simulink model "OpenLoopFreqResponse"  (R2015a)
settings: Solver=FixedStepDiscrete  SolverMode=SingleTasking  StartTime=0.0  StopTime=inf  FixedStep=Ts  RelTol=1e-3
InitFcn:
  | Ts = 0.010;
libraries: arduinolib x2, THLlib x2
settings Model: ExtModeTrigDuration=2  Creator=Carion  LastModifiedBy=SystemsUser
settings OptimizationCC: OptimizeModelRefInitCode=on  LifeSpan=1
settings DebuggingCC: UnderspecifiedInitializationDetection=Classic  MergeDetectMultiDrivingBlocksExec=none  StateNameClashWarn=warning
settings HardwareCC: ProdBitPerInt=16  ProdBitPerPointer=8  ProdIntDivRoundTo=Zero  ProdEndianess=LittleEndian  ProdWordSize=8  ProdHWDeviceType=Atmel->AVR
settings RTWCC: SystemTargetFile=realtime.tlc  GenerateMakefile=off  TemplateMakefile=realtime.tmf  Description=Run on Target Hardware  RTWVerbose=off
settings ERTTargetCC: CombineOutputUpdateFcns=off  ExtModeTransport=3  ExtModeMexFile=ext_serial_win32_comm  ExtModeMexArgs=0 1 9600  ERTSrcFileBannerTemplate=realtime_code_template.cgt  ERTHdrFileBannerTemplate=realtime_code_template.cgt  ERTDataSrcFileTemplate=realtime_code_template.cgt  ERTDataHdrFileTemplate=realtime_code_template.cgt  ERTCustomFileTemplate=realtime_file_process.tlc

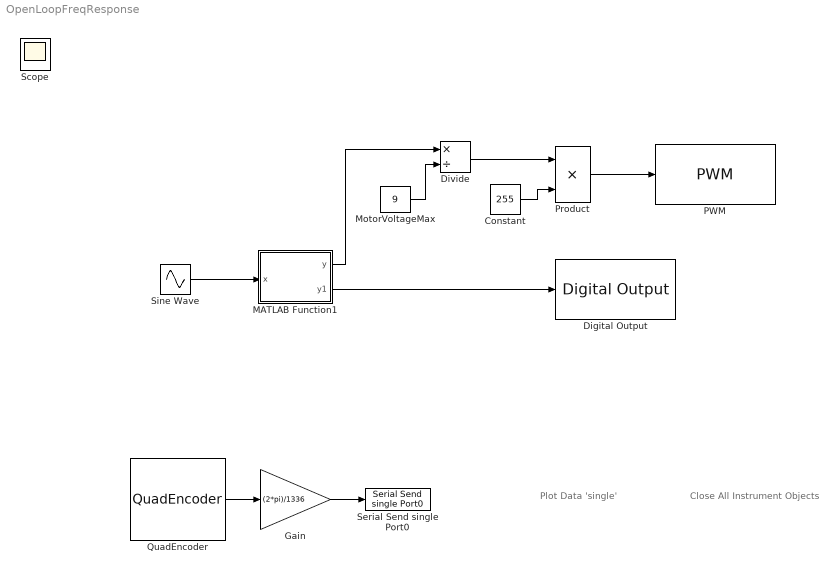
== system OpenLoopFreqResponse ==
  note: Close All
      | Instrument Objects
  note: Plot Data
      | 'single'
  Constant : Constant  Value=255
  Digital Output : arduinolib/Digital Output  pinNumber=4  blockPlatform=arduino
  Divide : Product  Inputs=*/  SampleTime=Ts
  Gain : Gain  Gain=(2*pi)/1336
  MATLAB Function1 : MATLAB Function  TreatAsAtomicUnit=on
  MotorVoltageMax : Constant  Value=9
  PWM : arduinolib/PWM  pinNumber=5  blockPlatform=arduino
  Product : Product  SampleTime=Ts
  QuadEncoder : THLlib/QuadEncoder
  Serial Send single Port0 : THLlib/Serial Send single Port0
  Sine Wave : Sin  Amplitude=4  Frequency=2*pi*.01  SampleTime=Ts
  Scope : Scope
  wires:
  Constant/1 -> Product/2
  Product/1 -> PWM/1
  MotorVoltageMax/1 -> Divide/2
  Divide/1 -> Product/1
  MATLAB Function1/2(y1) -> Digital Output/1
  Sine Wave/1 -> MATLAB Function1/1(x)
  QuadEncoder/1 -> Gain/1
  MATLAB Function1/1(y) -> Divide/1
  Gain/1 -> Serial Send single Port0/1

== matlab function OpenLoopFreqResponse/MATLAB Function1 ==
  data: x input; y output; y1 output
function [y,y1] = fcn(x)
%#codegen
if x>=0
    y=x;
    y1=0;
else
    y=-x;
    y1=1;
end
